simulink model "main_lowpath"  (R2026a)
settings: Solver=VariableStepAuto  StopTime=15  FixedStep=params.MPC.dt  RelTol=1e-2
values from neighbouring files (symbols this model uses):
  P_initial = params.Pd_initial + params.Pcm_initial    [setup_lowpath.m]
undefined symbols (not defined in the file or in its folder): params, Ref
(part 2 of 2)

== matlab function main_lowpath/Air_supply_system1 ==
  data: x input; Vcm input; dx output size=4; Ifc input; params parameter; Ref parameter
function dx = Air_supply_4d(x,Vcm,Ifc,params,Ref)
%saturation
% if Vcm < 0  
%    Vcm = 150;
% elseif Vcm > params.Vcm_u/Ref.Vcm 
%    Vcm = params.Vcm_u/Ref.Vcm ;
% end
% 
% if Ifc < 0 
%     Ifc = 0;
% elseif Ifc > 2.2*params.Afc/Ref.Ifc   
%     Ifc = 2.2*params.Afc/Ref.Ifc;
% end

if params.c11/(x(1)+x(2)+params.c2/Ref.pres)>params.c19*Ref.pres
    dx = Air_supply_case1(x,[Vcm;Ifc],[0;0]);
else
    dx = Air_supply_case2(x,[Vcm;Ifc],[0;0]);
end

% x = x./[Ref.x];
% Vcm = Vcm./Ref.Vcm;
% Ifc = Ifc./Ref.Ifc;
% dx = dx.*[Ref.x];

% R_= 8.314;  %Universal gas constant
% patm = 1.01325e5;  %Atomospheric pressure
% psat = 4.736e4;  %Saturation pressure 353K 
% Tatm = 298.15;   %Atmosphric temperature
% Tst = 353.15;    %Temperature of fuel-cell stack 
% Mo2 = 32e-3; %Molar mass of oxygen
% Mn2 = 28e-3; %Molar mass of nitrogen
% Mv = 18.02e-3; %Molar mass of vapour
% Maatm = 28.97e-3; %Molar mass of atmospheric air
% gam = 1.4;  %Air specific heat ratio
% Cp = 1004;   %Air specific ratio
% F = 96487;  %Faraday's constant
% kt = 0.0153;    %motor constant
% kv = 0.0153;    %motor constant
% Rcm = 0.82;    %motor constant
% Jcp = 5e-5;     %compressor and motor interia
% eata_cp = 0.80; %Compressor efficiency
% eata_cm = 0.98; %Compressor motor mechanical efficiency
% n = 381;    %Number of cells in fuel-cell stack
% Afc = 280;   %Fuel-cell active area (cm^2)
% Vsm = 0.02;     %Supply manifold volume
% Vca = 0.01;     %Single stack cathode volume
% kcain = 0.3629e-5; %Cathode inlet orifice
% tm = 1.275e-4;
% Cd = 0.0124;    %Cathode output throttle discharge cofficient
% At = 0.002;     %Cathode output throttle area
% phi_atm = 0.5;  %Average ambient air relative humidity
% yo2atm = 0.21;  %Oxygen molar ratio at cathode inlet
% xo2atm =yo2atm*Mo2/(yo2atm*Mo2+(1-yo2atm)*Mn2); %Oxygen mass fraction at cathode inlet
% watm =Mv/(yo2atm*Mo2+(1-yo2atm)*Mn2)*(phi_atm*psat/(patm-phi_atm*psat)); %Humidity ratio of inlet air
% Kapper = sqrt(mean([Mo2^2,Mn2^2,Mv^2]));
% Vcm_u = 300;
% 
% c1 = (R_*Tst*kcain)/(Mo2*Vca)*(xo2atm/(1+watm));
% c2 = psat;
% c3 = R_*Tst/Vca;
% c4 = Mo2;
% c5 = Mn2;
% c6 = Mv*psat;
% c7 = (R_*Tst*n)/(4*Vca*F);
% c8 = (R_*Tst*kcain)/(Mn2*Vca)*((1-xo2atm)/(1+watm));
% c9 = eata_cm*kt*kv/(Jcp*Rcm);
% c10 = Cp*Tatm/(Jcp*eata_cp);
% c11 = patm;
% c12 = (gam-1/gam);
% c13 = eata_cm*kt/(Jcp*Rcm);
% c14 = R_*Tatm/(Maatm*Vsm);
% c15 = 1/eata_cp;
% c16 = kcain;
% c17 = (Cd*At)/sqrt(R_*Tst)*sqrt(2*gam/(gam-1));
% c18 = 1/gam;
% c19 = (2/(gam+1))^(gam/(gam-1));
% c20 = (Cd*At)/sqrt(R_*Tst)*gam^(1/2)*(2/(gam+1))^((gam+1)/2*(gam-1));
% c21 = 1/Rcm;
% c22 = kv;
% c23 = kcain*xo2atm/(1+watm);
% c24 = n*Mo2/(4*F);
% 
% 
% if c11/(x(1)+x(2)+c2) > c19
% dx = [
%     c1*(-x(1)-x(2)+x(4)-c2)-(c3*x(1)*psi_case1(x,c2,c11,c12,c17,c18,c19,c20))/(c4*x(1)+c5*x(2)+c6)-c7*Ifc;
%     c8*(-x(1)-x(2)+x(4)-c2)-(c3*x(2)*psi_case1(x,c2,c11,c12,c17,c18,c19,c20))/(c4*x(1)+c5*x(2)+c6);
%     -c9*x(3)-(c10./x(3))*((x(4)./c11).^c12-1)*Weight_flow(x(3),x(4))+c13*Vcm;
%     c14*(1+c15*((x(4)./c11)^c12-1))*(Weight_flow(x(3),x(4))-c16*(-x(1)-x(2)+x(4)-c2))];
% else
% 
% dx =  [
%     c1*(-x(1)-x(2)+x(4)-c2)-(c3*x(1)*psi_case2(x,c2,c11,c12,c17,c18,c19,c20))/(c4*x(1)+c5*x(2)+c6)-c7*Ifc;
%     c8*(-x(1)-x(2)+x(4)-c2)-(c3*x(2)*psi_case2(x,c2,c11,c12,c17,c18,c19,c20))/(c4*x(1)+c5*x(2)+c6);
%     -c9*x(3)-(c10./x(3))*((x(4)./c11).^c12-1)*Weight_flow(x(3),x(4))+c13*Vcm;
%     c14*(1+c15*((x(4)./c11)^c12-1))*(Weight_flow(x(3),x(4))-c16*(-x(1)-x(2)+x(4)-c2))];
% end
% 
% 
% 
% 
% %%%%%%%%%%%%%%%%%%%%%%%%%%%%%%%%%%%%%%%%%%%%%%%%%%%%%%%%%%%%%%%%%%%%%%%%%%%%
% 
% end
% 
% function psi = psi_case1(x,c2,c11,c12,c17,c18,c19,c20)
% psi = c17*(x(1)+x(2)+c2)*(c11/(x(1)+x(2)+c2))^c18*sqrt(1-(c11/(x(1)+x(2)+c2))^c12);
% end
% 
% function psi = psi_case2(x,c2,c11,c12,c17,c18,c19,c20)
% psi = c20*(x(1)+x(2)+c2);
% end

== matlab function main_lowpath/Battery2 ==
  data: Ib input; Batt input; dBatt output; Ref parameter
function dBatt = fcn(Ib,Batt,Ref)
% if Ib <-36/Ref.Ib
%     Ib = -36/Ref.Ib;
% elseif Ib > 36/Ref.Ib
%     Ib = 36/Ref.Ib;
% end
Ib = Ib/15; %pararel 15

dBatt = Battery(Batt,Ib,0);
% Vsoc = Batt(1);
% Vs = Batt(2);
% Vf = Batt(3);

% Cb = 3060;
% SOC = Vsoc*100;
% Rsd = 10e9;
% Rs = 0.3208*exp(-29.14*SOC) +0.04669;
% Cs = -752.9*exp(-13.51*SOC) + 703.6;
% Rf = 6.603*exp(-155.2*SOC) +0.04984;
% Cf = -6056*exp(-27.12*SOC) + 4475;
% 
% 
% dVsoc = -Vsoc/(Rsd*Cb)-Ib/Cb;
% dVs = -Vs/(Rs*Cs)+Ib/Cs;
% dVf = -Vf/(Rf*Cf)+Ib/Cf;
% 
% dBatt = [dVsoc;dVs;dVf];

== matlab function main_lowpath/LowPath Filter1 ==
  data: P output; Pd output; Pd_str input; de output; Pcm input; e input; params parameter
function [P,Pd,de] = fcn(Pd_str,Pcm,e, params)
w_n = 1;
zeta = 1;
% シミュレーション時間が切り悪いときなにかする必要あり
Pd  = Pd_str(1);
P = Pd + Pcm;
e1 = e(1);
e2 = e(2);

% 論文の式14
% % % % % % % % % % % % % % % % % % % % % % 
de1 = e2;
de2 = -w_n^2*e1 -2*w_n*zeta*e2 + w_n^2*P; % 最後の項はzetaでなくw_n?
% % % % % % % % % % % % % % % % % % % % % % 
de = [de1;de2];
end

== matlab function main_lowpath/MATLAB Function10 ==
  data: e input; Pb_bar output; P input
function Pb_bar = fcn(e, P)

Pfc_bar = e(1);
Pb_bar = P - Pfc_bar; % P = Pd + Pcm
end

== matlab function main_lowpath/fuel_cel_systeml1 ==
  data: x input; Vcm input; Ifc input; Vfc output; Pcm output; params parameter
function [Vfc,Pcm] = fcn(x,Vcm,Ifc,params)
Pcm = Vcm*(Vcm-params.kv*x(3))/(params.Rcm*params.eata_cm);
Tfc = params.Tst;
po2 = x(1);
pH2 = x(1)+x(2);


E = 1.229-0.85e-3*(Tfc-params.Tatm)+4.3085e-5*Tfc*(reallog(pH2/params.patm)+1/2*reallog(po2/params.patm));
v0 = 0.279-8.5e-4*(Tfc-params.Tatm)+4.308e-5*Tfc*(reallog((x(1)+x(2))/params.patm)+1/2*reallog(0.1173*(x(1)+x(2))/params.patm));
va = (-1.68e-5*Tfc+1.618e-2)*(1.01325*(po2/0.1173+params.psat)/params.patm)^2+(1.8e-4*Tfc-0.166)*(1.01325*(po2/0.1173+params.psat)/params.patm)+(-5.8e-4*Tfc+0.5736);
a1 = 10;
I = Ifc/params.Afc;
vact = v0+va*(1-exp(-a1*I));
b11 = 5.139e-3;
b12 = 3.26e-3;
b2 = 350;
mu_m = 14; % vapor 100%
sig_m = (b11*mu_m-b12)*exp(b2*(1/303-1/Tfc));
Rohm = params.tm/sig_m;
vohm = I*Rohm;

if (po2/0.1173+params.psat) < 2*params.patm
a2 = (7.16e-4*Tfc-0.622)*1.01325*(po2/0.1173+params.psat)/params.patm+(-1.45e-3*Tfc+1.68);
else 
a2 = (8.66e-5*Tfc-0.068)*1.01325*(po2/0.1173+params.psat)/params.patm+(-1.6e-4*Tfc+0.54);
end
Imax = 2.2;
a3 = 2;
vconc = I*(a2*I/Imax)^a3;

vfc = E-vact-vohm-vconc;
Vfc = vfc*params.n;

== matlab function main_lowpath/MATLAB Function11 ==
  data: Pb_bar input; Ib_bar output; Vb input
function Ib_bar = fcn(Pb_bar,Vb)

Ib_bar = Pb_bar/Vb;
end

== matlab function main_lowpath/MATLAB Function6 ==
  data: Batt input; Pb output; Ib input; Vb output; SOC output
function [Pb,Vb,SOC] = fcn(Batt,Ib)
Ib = Ib/15; %pararel
Vsoc = Batt(1);
Vs = Batt(2);
Vf = Batt(3);
SOC = Vsoc ;
Voc = -1.031*exp(-35*SOC)+3.685+0.2156*SOC-0.1178*SOC^2+0.3201*SOC^3;
R0 = 0.1562*exp(-24.37*SOC)+0.07446;
Vb = Voc-R0*Ib-Vs-Vf;
Ib = Ib*15;
Pb = Ib*Vb*12; %series 12

== matlab function main_lowpath/MATLAB Function8 ==
  data: Ib input; Pfc output; Vb input; P input
function Pfc = fcn(Ib,Vb,P)

Pb = Ib*Vb;
Pfc = P - Pb; % P = Pd + Pcm
end

== matlab function main_lowpath/MATLAB Function9 ==
  data: SOC input; Ib_bar input; Ib output
function Ib = fcn(SOC, Ib_bar)
% SOCによってはIb_barに調整を入れる
Ib = Ib_bar;
end

== matlab function main_lowpath/NMPC1 ==
  data: Ifc input; z_ref input; x input size=params.nx; u_bar input size=[params.nu,params.MPC.N]; du1 output size=params.nu; Pd input; K0 output size=[params.nu,params.nx]; u_bar output size=[params.nu,params.MPC.N]; params parameter; x_ output size=params.nx; Ref parameter; Smax input size=1; u_b input size=[params.nu,params.MPC.N]; u_b output size=[params.nu,params.MPC.N]; ub1 output size=[params.nu 1]; rammda input; rammda output
function [du1,K0,u_bar,x_,u_b,ub1,rammda] = ILQR(Ifc,z_ref,x,u_bar,Pd,params,Ref,Smax,u_b,rammda)
% function [du1,K0,u_bar,x_,u_b,ub1,Pb_bar,rammda, nominal_AL_Bus] = ILQR(x,u_bar,Pd,params,Ref,Smax,u_b,rammda)
%UNTITLED3 この関数の概要をここに記述
%   詳細説明をここに記述
du = u_bar-u_b;
% which discretization method
D_method = 'V';                 % D:difference, V:variational


%%%%%%%%%%%%%%%%%%%%%% MPC setting %%%%%%%%%%%%%%%%%%%%%%%%%%%%%%%%%%%%%%%%
% linesearch off:0 on:1
linesearch = 1;
tsp = params.MPC.dt;            % sampling period
N = 10;                         % number of horizon 
N_iter = params.N_iter;         % number of N_iter


nx = size(x,1);                 
nu = size(u_b,1);             
K0 = zeros(nu,nx);             
x_bar = zeros(nx,N+1);
x_opt = zeros(nx,N+1);
%%%%%%%%%%%%%%%%% Augumented Lagrangian setting %%%%%%%%%%%%%%%%%%%%%%%%%%%
nc = 7;
nc_i = params.nc_i;
Altro.mu = repmat(4e-4,nc,N+1);
Altro.I_mu = zeros(nc,(N+1)*nc);
Altro.rammda = rammda;
Altro.rammda = zeros(nc,N+1);
Altro.cmax = 1e-8;
Altro.phi = 2;
Value_c = ones(nc,N+1);

for i = 1:N_iter

     for ii = 1:N+1
         for jj = 1:nc
                if Value_c(jj,ii) < 0 && Altro.rammda(jj,ii) == 0 && jj <= nc_i
                    Altro.I_mu(jj,nc*(ii-1)+jj) = 0;
                else
                    Altro.I_mu(jj,nc*(ii-1)+jj) = Altro.mu(jj,ii);
                if Altro.mu(jj,ii)<=100
                    Altro.mu(jj,ii) = Altro.mu(jj,ii)*Altro.phi;
                end
                end

         end
    end

          %disp('AL--------------')
          %disp(i)

% 一旦コメントアウトしてみる
Ist = Ifc; %もともと入力u2,du2だったものを，Ist,dIstとして関数に代入する．duはノミナルとの差であり，今回はdIst=0として，u2+du2=Ifcとなるようにしている．
dIst = 0;
    [x_bar,A,B] = forwardpass(x,u_b,du,Ist,dIst,tsp,N,D_method,params,Ref);
    [du,K0] = backwardpass_Altro_e(x_bar,u_b,du,Ist,dIst,A,B,N,tsp,linesearch,Pd,params,Altro,Ref,Smax,z_ref,u_b);




    % [x_bar,A,B] = forwardpass_runge(x,u_b,du,tsp,N,D_method,params,Ref);
    % [du,x_opt, K0] = backwardpass_Altro_e_runge(x_bar,u_b,du,A,B,N,tsp,linesearch,Pd,params,Altro,Ref,Smax);
        for ii = 1:N+1

            if ii ~= N+1
                [x_bar(:,ii),du(:,ii)] = satulation(x_bar(:,ii),u_b(:,ii),du(:,ii));
                if (x_bar(1,:)/0.1173+params.psat/Ref.pres) < 2
                    Value_c(:,ii) = constraints_case1(x_bar(:,ii),u_b(:,ii),du(:,ii),Pd(ii),Smax);
                else
                    Value_c(:,ii) = constraints_case2(x_bar(:,ii),u_b(:,ii),du(:,ii),Pd(ii),Smax);
                end
            else
                [x_bar(:,ii),~] = satulation(x_bar(:,ii),u_b(:,ii-1),du(:,ii-1));
                if (x_bar(1,:)/0.1173+params.psat/Ref.pres) < 2
                    Value_c(:,ii) = constraints_case1(x_bar(:,ii),u_b(:,ii-1),du(:,ii-1),Pd(ii-1),Smax);
                else
                    Value_c(:,ii) = constraints_case2(x_bar(:,ii),u_b(:,ii-1),du(:,ii-1),Pd(ii-1),Smax);
                end
            end

            for jj = 1:nc

                if Value_c(jj,ii) < 0 && Altro.rammda(jj,ii) == 0 && jj <= nc_i
                    Altro.rammda(jj,ii) = max([Altro.rammda(jj,ii) + Altro.mu(jj,ii).*Value_c(jj,ii),0]);
                elseif jj>nc_i
                    Altro.rammda(jj,ii) = Altro.rammda(jj,ii) + Altro.mu(jj,ii).*Value_c(jj,ii);
                else
                end

            end
            % disp(Altro.rammda(:,ii))
        end
end
rammda = circshift(Altro.rammda,-1,2);
rammda(:,end) = rammda(:,end-1);

    % % % % % % % % % % % % % % % % % % % % % % % 
    % % rungeのとき以外に使うとエラーが出る
    % nominal_AL_Bus.u_b = u_b;
    % nominal_AL_Bus.du = du;
    % nominal_AL_Bus.K0 = K0;
    % nominal_AL_Bus.x_opt = x_opt; 
    % nominal_AL_Bus.rammda = rammda;
    % % % % % % % % % % % % % % % % % % % % % % % 



% 制御入力
x_ = x_bar(:,2);
% Pb_bar = Pb_fun(x_bar(:,1),u_b(:,1),du(:,1));
du1 = du(:,1);
ub1 = u_b(:,1);

% ノミナルな入力の更新
u_b = u_b+du;
u_bar = circshift(u_b,-1,2);
u_bar(:,end) = u_b(:,end-1);

== matlab function main_lowpath/fuel_cel_systeml2 ==
  data: x input; Vcm input; Ifc input; Vfc output; Pcm output; params parameter
function [Vfc,Pcm] = fcn(x,Vcm,Ifc,params)
Pcm = Vcm*(Vcm-params.kv*x(3))/(params.Rcm*params.eata_cm);
Tfc = params.Tst;
po2 = x(1);
pH2 = x(1)+x(2);


E = 1.229-0.85e-3*(Tfc-params.Tatm)+4.3085e-5*Tfc*(reallog(pH2/params.patm)+1/2*reallog(po2/params.patm));
v0 = 0.279-8.5e-4*(Tfc-params.Tatm)+4.308e-5*Tfc*(reallog((x(1)+x(2))/params.patm)+1/2*reallog(0.1173*(x(1)+x(2))/params.patm));
va = (-1.68e-5*Tfc+1.618e-2)*(1.01325*(po2/0.1173+params.psat)/params.patm)^2+(1.8e-4*Tfc-0.166)*(1.01325*(po2/0.1173+params.psat)/params.patm)+(-5.8e-4*Tfc+0.5736);
a1 = 10;
I = Ifc/params.Afc;
vact = v0+va*(1-exp(-a1*I));
b11 = 5.139e-3;
b12 = 3.26e-3;
b2 = 350;
mu_m = 14; % vapor 100%
sig_m = (b11*mu_m-b12)*exp(b2*(1/303-1/Tfc));
Rohm = params.tm/sig_m;
vohm = I*Rohm;

if (po2/0.1173+params.psat) < 2*params.patm
a2 = (7.16e-4*Tfc-0.622)*1.01325*(po2/0.1173+params.psat)/params.patm+(-1.45e-3*Tfc+1.68);
else 
a2 = (8.66e-5*Tfc-0.068)*1.01325*(po2/0.1173+params.psat)/params.patm+(-1.6e-4*Tfc+0.54);
end
Imax = 2.2;
a3 = 2;
vconc = I*(a2*I/Imax)^a3;

vfc = E-vact-vohm-vconc;
Vfc = vfc*params.n;

== matlab function main_lowpath/fuel_cel_systeml ==
  data: x input; Vcm input; Ifc input; Vfc output; Pcm output; params parameter
function [Vfc,Pcm] = fcn(x,Vcm,Ifc,params)
Pcm = Vcm*(Vcm-params.kv*x(3))/(params.Rcm*params.eata_cm);
Tfc = params.Tst;
po2 = x(1);
pH2 = x(1)+x(2);


E = 1.229-0.85e-3*(Tfc-params.Tatm)+4.3085e-5*Tfc*(reallog(pH2/params.patm)+1/2*reallog(po2/params.patm));
v0 = 0.279-8.5e-4*(Tfc-params.Tatm)+4.308e-5*Tfc*(reallog((x(1)+x(2))/params.patm)+1/2*reallog(0.1173*(x(1)+x(2))/params.patm));
va = (-1.68e-5*Tfc+1.618e-2)*(1.01325*(po2/0.1173+params.psat)/params.patm)^2+(1.8e-4*Tfc-0.166)*(1.01325*(po2/0.1173+params.psat)/params.patm)+(-5.8e-4*Tfc+0.5736);
a1 = 10;
I = Ifc/params.Afc;
vact = v0+va*(1-exp(-a1*I));
b11 = 5.139e-3;
b12 = 3.26e-3;
b2 = 350;
mu_m = 14; % vapor 100%
sig_m = (b11*mu_m-b12)*exp(b2*(1/303-1/Tfc));
Rohm = params.tm/sig_m;
vohm = I*Rohm;

if (po2/0.1173+params.psat) < 2*params.patm
a2 = (7.16e-4*Tfc-0.622)*1.01325*(po2/0.1173+params.psat)/params.patm+(-1.45e-3*Tfc+1.68);
else 
a2 = (8.66e-5*Tfc-0.068)*1.01325*(po2/0.1173+params.psat)/params.patm+(-1.6e-4*Tfc+0.54);
end
Imax = 2.2;
a3 = 2;
vconc = I*(a2*I/Imax)^a3;

vfc = E-vact-vohm-vconc;
Vfc = vfc*params.n;

== matlab function main_lowpath/MATLAB Function ==
  data: Batt input; Pb output; Ib input; Vb output
function [Pb,Vb] = fcn(Batt,Ib)
Ib = Ib/15; %pararel
Vsoc = Batt(1);
Vs = Batt(2);
Vf = Batt(3);
SOC = Vsoc ;
Voc = -1.031*exp(-35*SOC)+3.685+0.2156*SOC-0.1178*SOC^2+0.3201*SOC^3;
R0 = 0.1562*exp(-24.37*SOC)+0.07446;
Vb = Voc-R0*Ib-Vs-Vf;
Ib = Ib*15;
Pb = Ib*Vb*12; %series 12

== matlab function main_lowpath/NMPC ==
  data: Ifc input size=1; z_ref input size=1; x input size=[4 1]; u_bar input size=[1 10]; du1 output size=1; Pd input size=[10 1]; K0 output size=[1 4]; u_bar output size=[params.nu,params.MPC.N]; params parameter; Ref parameter; Smax input size=1; u_b input size=[1 10]; u_b output size=[params.nu,params.MPC.N]; ub1 output size=1; rammda input size=[7 11]; rammda output; sannso output size=1
function [du1,K0,u_bar,u_b,ub1,rammda,sannso] = ILQR(Ifc,z_ref,x,u_bar,Pd,params,Ref,Smax,u_b,rammda)
% function [du1,K0,u_bar,x_,u_b,ub1,Pb_bar,rammda, nominal_AL_Bus] = ILQR(x,u_bar,Pd,params,Ref,Smax,u_b,rammda)
%UNTITLED3 この関数の概要をここに記述
%   詳細説明をここに記述
du = u_bar-u_b;
% which discretization method
D_method = 'V';                 % D:difference, V:variational


%%%%%%%%%%%%%%%%%%%%%% MPC setting %%%%%%%%%%%%%%%%%%%%%%%%%%%%%%%%%%%%%%%%
% linesearch off:0 on:1
linesearch = 1;
tsp = params.MPC.dt;            % sampling period
N = 10;                         % number of horizon 
N_iter = params.N_iter;         % number of N_iter


nx = size(x,1);                 
nu = size(u_b,1);             
K0 = zeros(nu,nx);             
x_bar = zeros(nx,N+1);
x_opt = zeros(nx,N+1);
%%%%%%%%%%%%%%%%% Augumented Lagrangian setting %%%%%%%%%%%%%%%%%%%%%%%%%%%
nc = 7;
nc_i = params.nc_i;
Altro.mu = repmat(4e-4,nc,N+1);
Altro.I_mu = zeros(nc,(N+1)*nc);
Altro.rammda = rammda;
Altro.rammda = zeros(nc,N+1);
Altro.cmax = 1e-8;
Altro.phi = 2;
Value_c = ones(nc,N+1);

l_check = zeros(1,N+1);
Ist = 0;
for i = 1:N_iter

     for ii = 1:N+1
         for jj = 1:nc
                if Value_c(jj,ii) < 0 && Altro.rammda(jj,ii) == 0 && jj <= nc_i
                    Altro.I_mu(jj,nc*(ii-1)+jj) = 0;
                else
                    Altro.I_mu(jj,nc*(ii-1)+jj) = Altro.mu(jj,ii);
                if Altro.mu(jj,ii)<=100
                    Altro.mu(jj,ii) = Altro.mu(jj,ii)*Altro.phi;
                end
                end

         end
    end

          %disp('AL--------------')
          %disp(i)

    % l_check = zeros(1,11);

    Ist = Ifc; %もともと入力u2,du2だったものを，Ist,dIstとして関数に代入する．duはノミナルとの差であり，今回はdIst=0として，u2+du2=Ifcとなるようにしている．
    dIst = 0;
    % ode45
    % [x_bar,A,B] = forwardpass(x,u_b,du,Ist,dIst,tsp,N,D_method,params,Ref);
    % [du,x_opt,K0,l_check] = backwardpass_Altro_e(x_bar,u_b,du,Ist,dIst,A,B,N,tsp,linesearch,Pd,params,Altro,Ref,Smax,z_ref,u_b);

    % Runge-Kutta Method
    [x_bar,A,B] = forwardpass_runge(x,u_b,du,Ist,dIst,tsp,N,D_method,params,Ref);
    [du,x_opt,K0,l_check] = backwardpass_Altro_e_runge(x_bar,u_b,du,Ist,dIst,A,B,N,tsp,linesearch,Pd,params,Altro,Ref,Smax,z_ref,u_b);
    % % % % % % % % % % % % % % % % % % % % % % % % % % % % % % % % % % % % % % % % % % % % % % % % % % % % % % % % % 
    % % % % % % % % % % % % % % % % % % % % % % % % % % % % % % % % % % % % % % % % % % % % % % % % % % % % % % % % % 

    % satulation以前の，「状態，制御入力」をもとに酸素過剰率の計算をしてみる．
    % u_b_check = u_b+du;
    % % その瞬間における酸素過剰率の計算
    % % sannso = z_fun(x,ub1,du1);
    % 
    % % nominalにおける酸素過剰率の計算
    % sannso_array = zeros(1,N);
    % for i = 1:N
    %     sannso_array(i) = z_fun(x_bar(:,i),u_b(i),0);
    % end
    % 
    % % Jの計算
    % J_part_sannso = 0; % 変数の定義
    % for i = 1:N
    %     J_part_sannso = J_part_sannso + (sannso_array(i)-z_ref)^2*params.MPC.Qs;
    % end
    % J_part_u = sum(du*du.'*params.MPC.R);
    % disp('============= ILQR before saturation ==================')
    % disp([z_ref, z_fun(x_bar(:,ii),Ist,dIst)])
    % % disp('sannso')
    % % disp(sannso)
    % disp('sannso_array')
    % disp(sannso_array)
    % disp('J_part_sannso')
    % disp(J_part_sannso)
    % disp('J_part_u')
    % disp(J_part_u)
    % disp('l_check')
    % disp(l_check)

    % % % % % % % % % % % % % % % % % % % % % % % % % % % % % % % % % % % % % % % % % % % % % % % % % % % % % % % % % 
    % % % % % % % % % % % % % % % % % % % % % % % % % % % % % % % % % % % % % % % % % % % % % % % % % % % % % % % % % 





       
        for ii = 1:N+1

            if ii ~= N+1
                [x_bar(:,ii),du(:,ii)] = satulation(x_bar(:,ii),u_b(:,ii),du(:,ii),Ref);
                if (x_bar(1,ii)/0.1173+params.psat/Ref.pres) < 2
                    Value_c(:,ii) = constraints_case1(x_bar(:,ii),u_b(:,ii),du(:,ii),Pd(ii),Smax);
                else
                    Value_c(:,ii) = constraints_case2(x_bar(:,ii),u_b(:,ii),du(:,ii),Pd(ii),Smax);
                end
            else
                [x_bar(:,ii),~] = satulation(x_bar(:,ii),u_b(:,ii-1),du(:,ii-1),Ref);
                if (x_bar(1,ii)/0.1173+params.psat/Ref.pres) < 2
                    Value_c(:,ii) = constraints_case1(x_bar(:,ii),u_b(:,ii-1),du(:,ii-1),Pd(ii-1),Smax);
                else
                    Value_c(:,ii) = constraints_case2(x_bar(:,ii),u_b(:,ii-1),du(:,ii-1),Pd(ii-1),Smax);
                end
            end

            for jj = 1:nc

                if Value_c(jj,ii) < 0 && Altro.rammda(jj,ii) == 0 && jj <= nc_i
                    Altro.rammda(jj,ii) = max([Altro.rammda(jj,ii) + Altro.mu(jj,ii).*Value_c(jj,ii),0]);
                elseif jj>nc_i
                    Altro.rammda(jj,ii) = Altro.rammda(jj,ii) + Altro.mu(jj,ii).*Value_c(jj,ii);
                else
                end

            end
            % disp(Altro.rammda(:,ii))
        end
end
rammda = circshift(Altro.rammda,-1,2);
rammda(:,end) = rammda(:,end-1);

    % % % % % % % % % % % % % % % % % % % % % % % 
    % % rungeのとき以外に使うとエラーが出る
    % nominal_AL_Bus.u_b = u_b;
    % nominal_AL_Bus.du = du;
    % nominal_AL_Bus.K0 = K0;
    % nominal_AL_Bus.x_opt = x_opt; 
    % nominal_AL_Bus.rammda = rammda;
    % % % % % % % % % % % % % % % % % % % % % % % 



% 制御入力
x_ = x_bar(:,2);
% Pb_bar = Pb_fun(x_bar(:,1),u_b(:,1),du(:,1));
du1 = du(:,1);
ub1 = u_b(:,1);

% ノミナルな入力の更新
u_b = u_b+du;
u_bar = circshift(u_b,-1,2);
u_bar(:,end) = u_b(:,end-1);

% その瞬間における酸素過剰率の計算
% sannso = z_fun(x,ub1,du1); %ここ引数を間違ってた
sannso = z_fun(x,Ist,0);

% % nominalにおける酸素過剰率の計算
% sannso_array = zeros(1,N);
% for i = 1:N
%     % sannso_array(i) = z_fun(x_bar(:,i),u_b(i),0);
%     sannso_array(i) = z_fun(x_bar(:,i),Ist,0);
% end
% 
% % Jの計算
% J_part_sannso = 0; % 変数の定義
% for i = 1:N
%     J_part_sannso = J_part_sannso + (sannso_array(i)-z_ref)^2*params.MPC.Qs;
% end
% J_part_u = sum(du*du.'*params.MPC.R);
% 
% % if 文でsimulink実行時に隠す
% if coder.target('MATLAB')
%     % ここに追加したデバッグ用のコードを書く
%     disp('============= ILQR after saturation ==================')
%     % disp('sannso')
%     % disp(sannso)
%     disp('sannso_array')
%     disp(sannso_array)
%     disp('J_part_sannso')
%     disp(J_part_sannso)
%     disp('J_part_u')
%     disp(J_part_u)
%     disp('l_check')
%     disp(l_check)
    % disp('================================================')
end


% backwardpassのなかではz_funは大体2の値をかえす
% backwardpassのあとにz_funの値をみたらもう1になってしまっていた．
% backwardpassの中でもうすでにx_bar,duの値が修正されている可能性がある．
%

== matlab function main_lowpath/IP_ILQR_controller_test/IP-ILQR ==
  data: x input size=params.nx; u_bar input size=[params.nu,params.MPC.N]; u1 output size=params.nu; Pd input; K0 output size=[params.nu,params.nx]; u_bar output size=[params.nu,params.MPC.N]; params parameter; x_bar_next output size=params.nx; Ref parameter; Smax input; Pb_bar output size=1; s_bar input; s_opt output; nominal_IP_Bus output Bus: nominal_IP_Bus
 function [u1,K0,u_bar, x_bar_next, Pb_bar, s_opt, nominal_IP_Bus] = ILQR(x,u_bar,Pd,params,Ref,Smax,s_bar)

% which discretization method
% D:difference, V:variational
D_method = 'D or V';
if params.D_method == 1
    D_method = 'D';       % 1:difference, 0:
    disp(D_method)
elseif params.D_method == 0
    D_method = 'V';
     % disp(D_method)
end

% 前の時間ステップからの時刻のずれを補正
u_bar(:,1:end-1) = u_bar(:,2:end);
u_bar(:,end)     = u_bar(:,end-1);
du = zeros(size(u_bar));

s_bar(:,1:end-1)   = s_bar(:,2:end);
s_bar(:,end)       = s_bar(:,end-1);

%%%%%%%%%%%%%%%%%%%%%% MPC setting %%%%%%%%%%%%%%%%%%%%%%%%%%%%%%%%%%%%%%%%
% linesearch off:0 on:1
linesearch = params.lineserch;
tsp = params.MPC.dt;            % sampling period
N = 10;                         % number of horizon 
N_iter = params.N_iter_IP;         % number of N_iter_IP

nx = size(x,1);                 
nu = size(u_bar,1);

K0 = zeros(nu,nx);             
x_bar = zeros(nx,N+1);
x_opt = zeros(nx,N+1);
du_IP = zeros(nu,N);
K0_IP = zeros(nu,nx);
x_opt_IP = zeros(nx,N+1);
du_opt = zeros(nu,N);
Qu = zeros(size(u_bar));
Qu_hat = zeros(size(u_bar));


%%%%%%%%%%%%%%%%% Interior Point setting %%%%%%%%%%%%%%%%%%%%%%%%%%%%%%%%%
mu = params.MPC.mu;
mu_iter = params.mu_iter;
mu_decrease_rate = params.mu_decrease_rate;

disp('==========================0.05s')



s_opt = zeros(size(s_bar));
c    = zeros(size(s_bar));


% 各μにおけるc,r,sの値を保存する変数
c_mu = zeros(size(c,1),size(c,2),mu_iter);  
r_mu = zeros(size(c_mu,1),size(c_mu,2),mu_iter);
s_mu = zeros(size(r_mu));
Qu_mu = zeros(size(u_bar,1),size(u_bar,2),mu_iter);
Qu_hat_mu = zeros(size(u_bar,1),size(u_bar,2),mu_iter);
%%%%%%%%%%%%%%%%% Iteration %%%%%%%%%%%%%%%%%%%%%%%%%%%%%%%%%%%%%%%%%%%%%%%
ls_gamma = 1;

for j = 1:mu_iter
   for i = 1:N_iter
        % disp('--------------') 
        if any(x_bar(1,:) < 0)
           disp(u_bar+du)
           disp(x_bar)
        end
   
        [x_bar,A,B]    = forwardpass_runge(x, u_bar, du, tsp, N, D_method,params,Ref);
        [du_opt, x_opt,s_opt,K0,ls_gamma,r] = backwardpass_IP_Quu_reg(x_bar, u_bar, du, s_bar,A,B,N,tsp,ls_gamma,Pd,params,mu,Ref,Smax);
        
        del_du = du_opt -du;
        du = du_opt;
        
        % =================================================================
        %　muの更新　
        % |F(w,s)| < 0.2*mu でN_iter の終了

        [r,Qu,Qu_hat] = F_wmu(x_opt,u_bar,du_opt,s_opt,A,B,N,Pd,params,mu,Ref,Smax);
        

        r_max = max(max(abs(r)));
        Qu_max = max(max(abs(Qu)));
        F_max = max(r_max,Qu_max);


        if r_max < mu(1)/5 && Qu_max < 1
            disp('r_max < mu/5')
            disp([j,i])
            disp([r_max,mu(1)/5])
            disp(r)
            disp(Qu)
            % Quの値があまりにも大きい場合はbreakしないようにしたい
            break
        % else
            % disp('r_max > mu/5')
            % disp([j,i])
            % disp([r_max,mu(1)/5])
            % disp(r)
        end

        % if F_max < mu(1)/5
        %     disp('F(w,mu) < mu/5')
        %     disp([j,i])
        %     disp([F_max,mu(1)/5])
        %     break
        % else
        %     disp([j,i])
        %     %disp([Qu_max,r_max])
        %     disp(del_du)
        %     disp(max(max(abs(Qu))))
        % 
        %     % if r_max > mu(1)/5
        %     %     disp('r_max > mu(1)/5')
        %     %     disp([r_max,mu(1)/5])
        %     % end
        %     % if Qu_max > mu(1)/5
        %     %     disp('Qu_max > mu(1)/5')
        %     %     disp([Qu_max,mu(1)/5])
        %     % end
        % end
        % =================================================================
   end

   
    %　各muでの r=s*c+muの計算
    for ii = 1:N
        if (x_opt(1,ii)/0.1173+params.psat/Ref.pres) < 2    
             c(:,ii) = constraints_case1(x_opt(:,ii),u_bar(:,ii),du_opt(:,ii),Pd(ii),Smax);
        else
             c(:,ii) = constraints_case2(x_opt(:,ii),u_bar(:,ii),du_opt(:,ii),Pd(ii),Smax);
        end
    end

    for ii = 1:N
        r_mu(:,ii,j)   = s_opt(:,ii).*c(:,ii)+mu;
        %r_mu(:,ii,j)   = s_opt(:,ii).*c(:,ii);
    end
    
    %  === mu毎における値の保存 ===
    c_mu(:,:,j) = c;
    s_mu(:,:,j) = s_opt;
    Qu_mu(:,:,j) = Qu;
    Qu_hat_mu(:,:,j) = Qu_hat;
    % ============================
    
    % disp(j)
    % disp(mu')
    % disp(c)
    % disp(s_opt)
    % disp(r_mu(:,:,j))
    
    % mu = mu./mu_decrease_rate;
    mu = mu/5;
    %mu(14:15) = mu(14:15)/25; 
end
% % % % % % % % % % % % % % % % % % % % % % % % % % % % % % % % % % % % % % 

Pb_bar = Pb_fun(x_bar(:,1),u_bar(:,1),du(:,1));
u1    = u_bar(:,1) + du(:,1); 
u_bar = u_bar + du;
x_bar_next = x_opt(:,2);




nominal_IP_Bus.u_b = u_bar;
nominal_IP_Bus.du = du;
nominal_IP_Bus.K0 = K0;
nominal_IP_Bus.x_opt = x_opt;
nominal_IP_Bus.s = s_opt;
nominal_IP_Bus.c = c;
nominal_IP_Bus.Qu = Qu;
nominal_IP_Bus.Qu_hat = Qu_hat;
nominal_IP_Bus.r = r_mu(:,:,end); % r_muはmuごとのrの値が入っている．その最後の値（イテレーションの最後）を保存
end
